simulink model "exp04"  (R2020b)
settings: Solver=VariableStepAuto  StartTime=0.0  StopTime=10.0  RelTol=1e-3
settings Model: Creator=1  LastModifiedBy=1

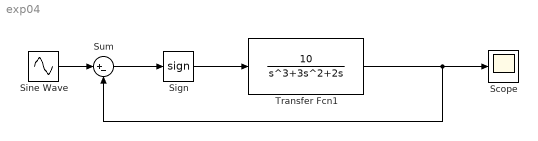
== system exp04 ==
  Scope : Scope
  Sign : Signum
  Sine Wave : Sin  SampleTime=0
  Sum : Sum  Inputs=|+-
  Transfer Fcn1 : TransferFcn  Numerator=[0 10]  Denominator=[1 3 2 0]
  wires:
  Sign/1 -> Transfer Fcn1/1
  Transfer Fcn1/1 -> Scope/1, Sum/2
  Sum/1 -> Sign/1
  Sine Wave/1 -> Sum/1
